simulink model "Wheelspeed_Sensor"  (R2025b)
settings: Solver=FixedStepAuto  StartTime=0.0  StopTime=10.0  FixedStep=0.00002  RelTol=1e-3
libraries: simulink x1
settings Model: Creator=finneinhoff  LastModifiedBy=finneinhoff

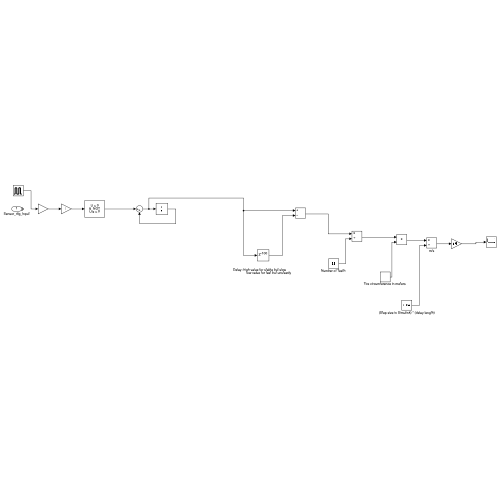
[thumbnail: Simulink's stored preview of the top-level diagram]
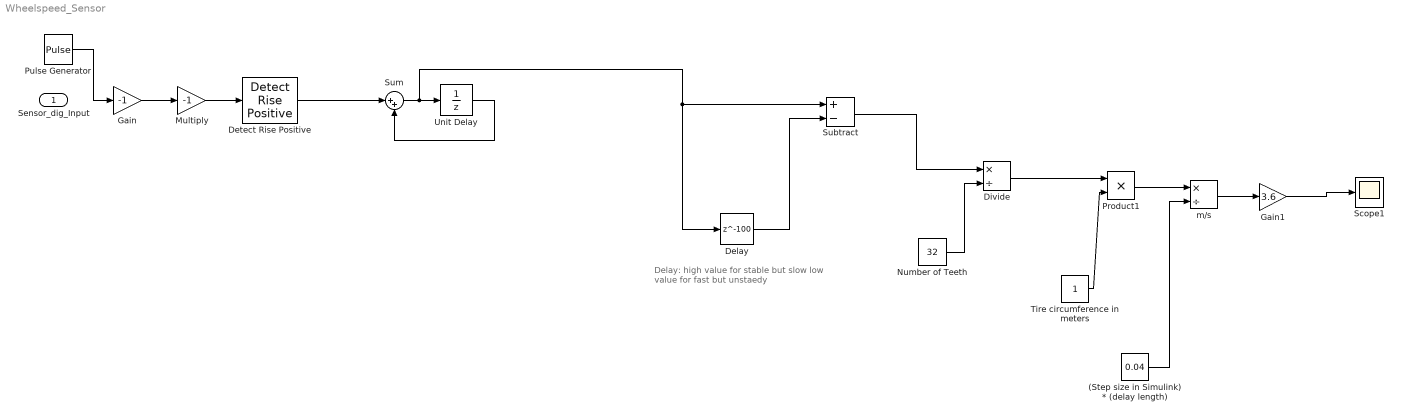
== system Wheelspeed_Sensor ==
  note: Delay: high value for stable but slow
      | 		low value for fast but unstaedy
  Sensor_dig_Input : Inport
  (Step size in Simulink) * (delay length) : Constant  Value=0.04
  Delay : Delay  DelayLength=100
  Detect Rise Positive : simulink/Logic and Bit Operations/Detect Rise Positive  vinit=0  OutDataTypeStr=uint8
  Divide : Product  Inputs=*/
  Gain : Gain  Gain=-1
  Gain1 : Gain  Gain=3.6
  Multiply : Gain  Gain=-1
  "Number of Teeth " : Constant  Value=32
  Product1 : Product
  Pulse Generator : DiscretePulseGenerator  PulseType=Time based  Period=0.00144  PulseWidth=50
  Scope1 : Scope
      settings: ActiveDisplayYMinimum=2.4319227132049517  ActiveDisplayYMaximum=5.9475477132049521
  Subtract : Sum  Inputs=+-
  Sum : Sum  Inputs=|++
  "Tire circumference in meters " : Constant
  Unit Delay : UnitDelay  SampleTime=-1  HasFrameUpgradeWarning=on
  m/s : Product  Inputs=*/
  wires:
  Gain/1 -> Multiply/1
  Multiply/1 -> Detect Rise Positive/1
  Detect Rise Positive/1 -> Sum/1
  Sum/1 -> Delay/1, Subtract/1, Unit Delay/1
  Delay/1 -> Subtract/2
  Pulse Generator/1 -> Gain/1
  Subtract/1 -> Divide/1
  Unit Delay/1 -> Sum/2
  "Number of Teeth "/1 -> Divide/2
  Divide/1 -> Product1/1
  "Tire circumference in meters "/1 -> Product1/2
  Product1/1 -> m/s/1
  (Step size in Simulink) * (delay length)/1 -> m/s/2
  m/s/1 -> Gain1/1
  Gain1/1 -> Scope1/1
